simulink model "i_1metre"  (R2023a)
settings: Solver=FixedStepDiscrete  StartTime=0.0  StopTime=30  FixedStep=0.01  RelTol=1e-3
values from neighbouring files (symbols this model uses):
  ticksPerRot = 10    [robotParameters.m]
  wheelR = 0.034    [robotParameters.m]
undefined symbols (not defined in the file or in its folder): DiscIntNeverNeededParam
libraries: arduinolib x10, simulink x8, simulink_extras x1, mobileRoboticsTrainingLib x1
settings Model: SimulationMode=external  ExtModeTrigDuration=2  Creator=Boitumelo  LastModifiedBy=cameronclark
settings OptimizationCC: EnhancedBackFolding=on  PassReuseOutputArgsAs=Individual arguments  ZeroExternalMemoryAtStartup=off  ZeroInternalMemoryAtStartup=off  MaxStackSize=64  OptimizeBlockOrder=speed  DifferentSizesBufferReuse=on  OptimizationCustomize=off  EfficientTunableParamExpr=on
settings DebuggingCC: ParameterTunabilityLossMsg=error  UnconnectedInputMsg=warning  UnconnectedOutputMsg=warning  UnconnectedLineMsg=warning
settings HardwareCC: ProdBitPerPointer=32  ProdBitPerSizeT=32  ProdBitPerPtrDiffT=32  ProdLargestAtomicInteger=Long  ProdLargestAtomicFloat=Double  ProdWordSize=32  ProdHWDeviceType=ARM Compatible->ARM Cortex  UseEmbeddedCoderFeatures=off  UseSimulinkCoderFeatures=off
settings ModelReferenceCC: EnableRefExpFcnMdlSchedulingChecks=on
settings SFSimCC: MATLABDynamicMemAlloc=off
settings RTWCC: Description=Embedded Coder  SystemTargetFile=ert.tlc  HardwareBoard=Arduino Nano 33 IoT  TemplateMakefile=ert_default_tmf  Toolchain=Arduino ARM  BuildConfiguration=Faster Runs  DLArmComputeVersion=19.05
settings CodeAppCC: ForceParamTrailComments=on  IgnoreCustomStorageClasses=off  OperatorAnnotations=on  SimulinkDataObjDesc=on  SFDataObjDesc=on  InsertBlockDesc=on
settings ERTTargetCC: SupportContinuousTime=on  SupportNonInlinedSFcns=on  SupportVariableSizeSignals=on  ExtModeTransport=3  ExtModeStaticAlloc=on  ExtModeAutomaticAllocSize=off  ExtModeStaticAllocSize=8192  ExtModeMexFile=ext_xcp  ExtModeIntrfLevel=Level2 - Open

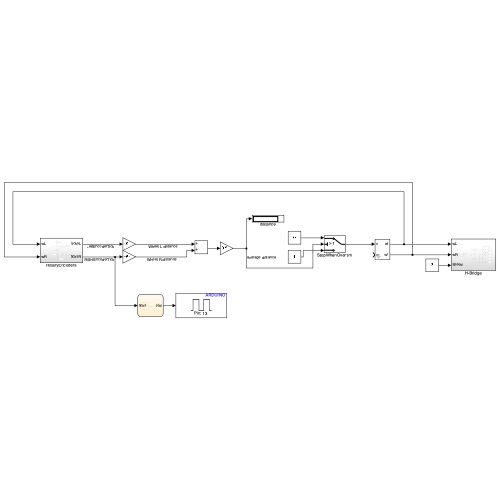
[thumbnail: Simulink's stored preview of the top-level diagram]
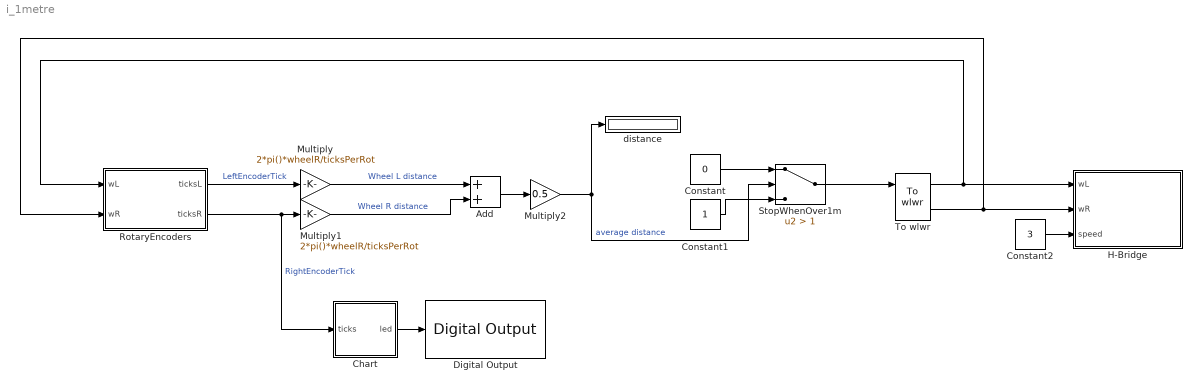
== system i_1metre ==
  Add : Sum
  Chart : Stateflow chart  TreatAsAtomicUnit=on
  Constant : Constant  Value=0
  Constant1 : Constant
  Constant2 : Constant  Value=3
  Digital Output : arduinolib/Digital Output  pinNumber=13  Direction=output  blockPlatform=arduino
  H-Bridge : Subsystem
  Multiply : Gain  Gain=2*pi()*wheelR/ticksPerRot
  Multiply1 : Gain  Gain=2*pi()*wheelR/ticksPerRot
  Multiply2 : Gain  Gain=0.5
  RotaryEncoders : Subsystem
  StopWhenOver1m : Switch  Criteria=u2 > Threshold  Threshold=1  SaturateOnIntegerOverflow=off  InputSameDT=off
  To wlwr : mobileRoboticsTrainingLib/To wlwr  axleLength=0.1  wheelR=0.05
  distance : Display
  wires:
  RotaryEncoders/1(ticksL) -> Multiply/1  "LeftEncoderTick"
  RotaryEncoders/2(ticksR) -> Chart/1(ticks), Multiply1/1  "RightEncoderTick"
  Constant/1 -> StopWhenOver1m/1
  Constant1/1 -> StopWhenOver1m/3
  StopWhenOver1m/1 -> To wlwr/1
  Multiply1/1 -> Add/2  "Wheel R distance"
  Multiply/1 -> Add/1  "Wheel L distance"
  Add/1 -> Multiply2/1
  Multiply2/1 -> distance/1, StopWhenOver1m/2  "average distance"
  To wlwr/1 -> RotaryEncoders/1(wL), H-Bridge/1(wL)
  To wlwr/2 -> RotaryEncoders/2(wR), H-Bridge/2(wR)
  Constant2/1 -> H-Bridge/3(speed)
  Chart/1(led) -> Digital Output/1

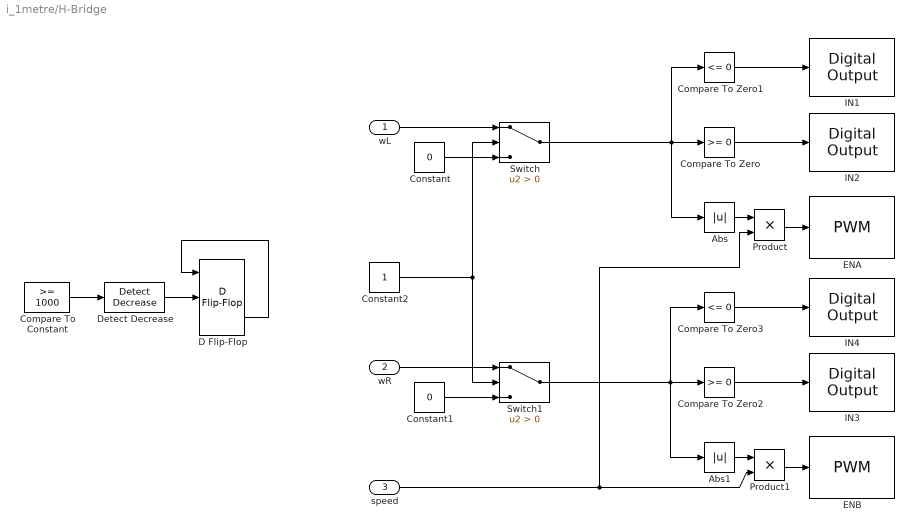
== system i_1metre/H-Bridge ==
  wL : Inport
  wR : Inport  Port=2
  speed : Inport  Port=3
  Abs : Abs  SaturateOnIntegerOverflow=off
  Abs1 : Abs  SaturateOnIntegerOverflow=off
  Compare To Constant : simulink/Logic and Bit Operations/Compare To Constant  relop=>=  const=1000  OutDataTypeStr=boolean
  Compare To Zero : simulink/Logic and Bit Operations/Compare To Zero  relop=>=  OutDataTypeStr=boolean
  Compare To Zero1 : simulink/Logic and Bit Operations/Compare To Zero  relop=<=  OutDataTypeStr=boolean
  Compare To Zero2 : simulink/Logic and Bit Operations/Compare To Zero  relop=>=  OutDataTypeStr=boolean
  Compare To Zero3 : simulink/Logic and Bit Operations/Compare To Zero  relop=<=  OutDataTypeStr=boolean
  Constant : Constant  Value=0
  Constant1 : Constant  Value=0
  Constant2 : Constant
  D Flip-Flop : simulink_extras/Flip Flops/D Flip-Flop
  Detect Decrease : simulink/Logic and Bit Operations/Detect Decrease  vinit=0.0  OutDataTypeStr=boolean
  ENA : arduinolib/PWM  pinNumber=4  frequencyType=Default  desiredFrequency=490.2  achievableFrequency=490.2
  ENB : arduinolib/PWM  pinNumber=5  frequencyType=Default  desiredFrequency=490.2  achievableFrequency=490.2
  IN1 : arduinolib/Digital Output  pinNumber=2  Direction=output  blockPlatform=arduino
  IN2 : arduinolib/Digital Output  pinNumber=3  Direction=output  blockPlatform=arduino
  IN3 : arduinolib/Digital Output  pinNumber=7  Direction=output  blockPlatform=arduino
  IN4 : arduinolib/Digital Output  pinNumber=6  Direction=output  blockPlatform=arduino
  Product : Product
  Product1 : Product
  Switch : Switch  Criteria=u2 > Threshold  SaturateOnIntegerOverflow=off  InputSameDT=off
  Switch1 : Switch  Criteria=u2 > Threshold  SaturateOnIntegerOverflow=off  InputSameDT=off
  wires:
  Compare To Zero/1 -> IN2/1
  Compare To Zero1/1 -> IN1/1
  Abs/1 -> Product/1
  wL/1 -> Switch/1
  Product/1 -> ENA/1
  Abs1/1 -> Product1/1
  Product1/1 -> ENB/1
  Compare To Zero2/1 -> IN3/1
  Compare To Zero3/1 -> IN4/1
  speed/1 -> Product/2, Product1/2
  Switch/1 -> Abs/1, Compare To Zero1/1, Compare To Zero/1
  Constant/1 -> Switch/3
  ? -> Compare To Constant/1
  Compare To Constant/1 -> Detect Decrease/1
  Constant1/1 -> Switch1/3
  Switch1/1 -> Compare To Zero2/1, Abs1/1, Compare To Zero3/1
  wR/1 -> Switch1/1
  Detect Decrease/1 -> D Flip-Flop/2
  D Flip-Flop/2 -> D Flip-Flop/1
  Constant2/1 -> Switch1/2, Switch/2

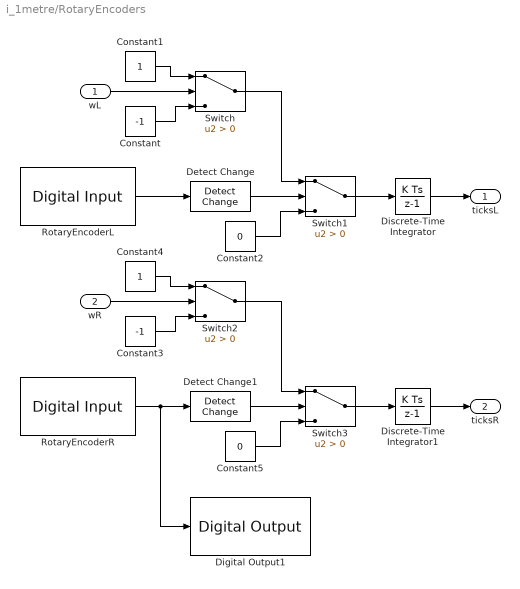
== system i_1metre/RotaryEncoders ==
  wL : Inport
  wR : Inport  Port=2
  Constant : Constant  Value=-1
  Constant1 : Constant
  Constant2 : Constant  Value=0
  Constant3 : Constant  Value=-1
  Constant4 : Constant
  Constant5 : Constant  Value=0
  Detect Change : simulink/Logic and Bit Operations/Detect Change  vinit=0  OutDataTypeStr=boolean
  Detect Change1 : simulink/Logic and Bit Operations/Detect Change  vinit=0  OutDataTypeStr=boolean
  Digital Output1 : arduinolib/Digital Output  pinNumber=10  Direction=output  blockPlatform=arduino
  Discrete-Time Integrator : DiscreteIntegrator  SampleTime=-1  ICPrevOutput=DiscIntNeverNeededParam  ICPrevScaledInput=DiscIntNeverNeededParam
  Discrete-Time Integrator1 : DiscreteIntegrator  SampleTime=-1  ICPrevOutput=DiscIntNeverNeededParam  ICPrevScaledInput=DiscIntNeverNeededParam
  RotaryEncoderL : arduinolib/Digital Input  pinNumber=8  mode=Default  Direction=input  SampleTime=0.1  blockPlatform=arduino
  RotaryEncoderR : arduinolib/Digital Input  pinNumber=9  mode=Default  Direction=input  SampleTime=0.1  blockPlatform=arduino
  Switch{,1..3} (4 alike) : Switch  Criteria=u2 > Threshold  SaturateOnIntegerOverflow=off  InputSameDT=off
  ticksL : Outport
  ticksR : Outport  Port=2
  wires:
  RotaryEncoderL/1 -> Detect Change/1
  wL/1 -> Switch/2
  Constant1/1 -> Switch/1
  Constant/1 -> Switch/3
  Switch1/1 -> Discrete-Time Integrator/1
  Discrete-Time Integrator/1 -> ticksL/1
  Switch/1 -> Switch1/1
  Constant2/1 -> Switch1/3
  Switch3/1 -> Discrete-Time Integrator1/1
  Switch2/1 -> Switch3/1
  Constant4/1 -> Switch2/1
  Constant5/1 -> Switch3/3
  Detect Change1/1 -> Switch3/2
  Constant3/1 -> Switch2/3
  wR/1 -> Switch2/2
  RotaryEncoderR/1 -> Digital Output1/1, Detect Change1/1
  Discrete-Time Integrator1/1 -> ticksR/1
  Detect Change/1 -> Switch1/2

== stateflow chart i_1metre/Chart ==
  state s
    during:
    if (mod(ticks,40) == 0)
    led = 1;
    end
  state ledOn
    exit:
    led = 0;
  (default) -> s
  s -> ledOn : [led==1]
  ledOn -> s : after(100, msec)
  data: led output; ticks input
